simulink model "convertidor_Opamp_Simulink"  (R2024b)
settings: Solver=VariableStepAuto  StartTime=0.0  StopTime=2  RelTol=1e-3
InitFcn:
  |     R1 = 5e6;   % 5M Ohms
  |     R2 = 5e6;   % 5M Ohms
  |     R3 = 5e6;   % 5M Ohms
  |     C1 = 100e-9; % 100nF
  |     C2 = 100e-9; % 100nF
settings Model: Creator=PC WHALE

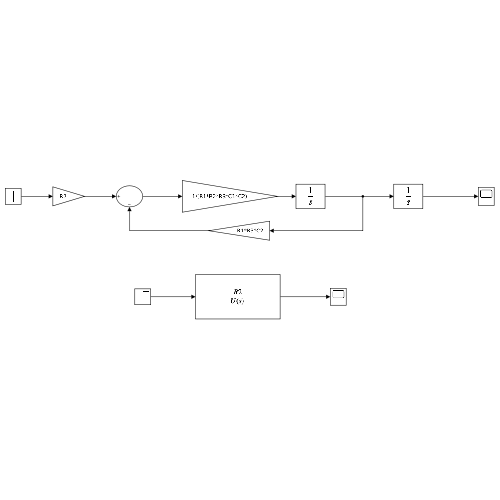
[thumbnail: Simulink's stored preview of the top-level diagram]
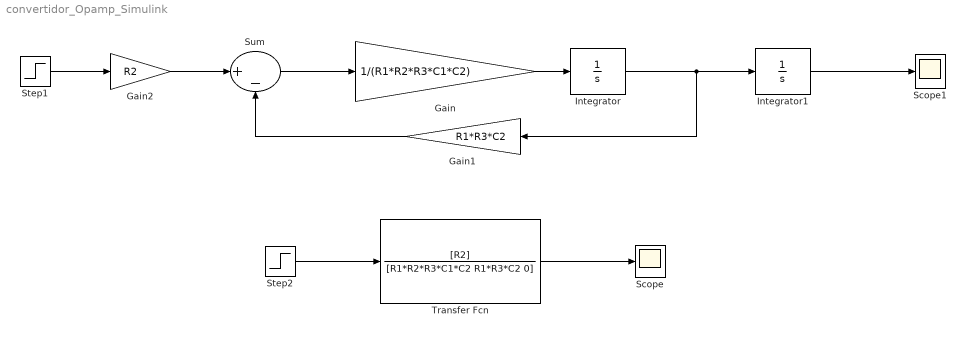
== system convertidor_Opamp_Simulink ==
  Gain : Gain  Gain=1/(R1*R2*R3*C1*C2)
  Gain1 : Gain  Gain=R1*R3*C2
  Gain2 : Gain  Gain=R2
  Integrator : Integrator
  Integrator1 : Integrator
  Scope : Scope
  Scope1 : Scope
  Step1 : Step  Time=0  After=5  SampleTime=0
  Step2 : Step  Time=0  After=5  SampleTime=0
  Sum : Sum  Inputs=|+-
  Transfer Fcn : TransferFcn  Numerator=[R2]  Denominator=[R1*R2*R3*C1*C2 R1*R3*C2 0]
  wires:
  Step1/1 -> Gain2/1
  Transfer Fcn/1 -> Scope/1
  Integrator/1 -> Integrator1/1, Gain1/1
  Gain/1 -> Integrator/1
  Sum/1 -> Gain/1
  Gain1/1 -> Sum/2
  Gain2/1 -> Sum/1
  Integrator1/1 -> Scope1/1
  Step2/1 -> Transfer Fcn/1
